simulink model "motor"  (R2015a)
settings: Solver=ode5  StartTime=0.0  StopTime=10  FixedStep=0.001  MaxStep=0.  RelTol=1e-3
undefined symbols (not defined in the file): sigbuilder_block
settings Model: Creator=Fares  LastModifiedBy=Fares

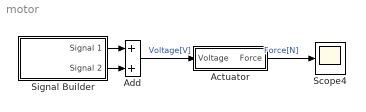
== system motor ==
  Actuator : Subsystem
  Add : Sum
  Scope4 : Scope
      settings: SaveName=ScopeData4
  Signal Builder : Subsystem  Tag=STV Subsys  LoadFcn=sigbuilder_block('load');  StartFcn=sigbuilder_block('start');  StopFcn=sigbuilder_block('stop');  ClipboardFcn=sigbuilder_block('clipboard');  mask(Sigbuilder block){}
      mask help: Simulink:masks:SigbuilderBlock_MD
      mask init:
      | if ~strcmp(get_param(bdroot(gcbh),'SimulationStatus'),'stopped') tuvar = sigbuilder_block('maskInit'); end
      settings: CopyFcn=sigbuilder_block('copy');  DeleteFcn=sigbuilder_block('delete');  ModelCloseFcn=sigbuilder_block('modelClose');  PreSaveFcn=sigbuilder_block('preSave');  PauseFcn=sigbuilder_block('pause');  ContinueFcn=sigbuilder_block('continue');  NameChangeFcn=sigbuilder_block('namechange');  OpenFcn=sigbuilder_block('open',[437.6 199.2 550.4 400 ]);  CloseFcn=sigbuilder_block('close');
      mask Display: plot(0, 0, 100, 100,[2, 2, 32, 32, 2], [68, 8, 8, 68, 68],[32, 2], [38, 38], [32, 19, 2],[53, 60, 44], [32, 17, 17, 2],[16, 16, 31, 31]);txt = getActiveGroup(gcbh);text(2, 100, txt,'verticalAlignment', 'top');
  wires:
  Actuator/1(Force) -> Scope4/1  "Force[N]"
  Signal Builder/1(Signal 1) -> Add/1
  Add/1 -> Actuator/1(Voltage)  "Voltage[V]"
  Signal Builder/2(Signal 2) -> Add/2

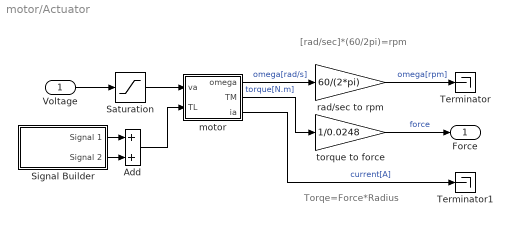
== system motor/Actuator ==
  note: Torqe=Force*Radius
  note: [rad/sec]*(60/2pi)=rpm
  Voltage : Inport
  Add : Sum
  Saturation : Saturate  UpperLimit=25  LowerLimit=-25
  Signal Builder : Subsystem  Tag=STV Subsys  LoadFcn=sigbuilder_block('load');  StartFcn=sigbuilder_block('start');  StopFcn=sigbuilder_block('stop');  ClipboardFcn=sigbuilder_block('clipboard');  mask(Sigbuilder block){}
      mask help: Simulink:masks:SigbuilderBlock_MD
      mask init:
      | if ~strcmp(get_param(bdroot(gcbh),'SimulationStatus'),'stopped') tuvar = sigbuilder_block('maskInit'); end
      settings: CopyFcn=sigbuilder_block('copy');  DeleteFcn=sigbuilder_block('delete');  ModelCloseFcn=sigbuilder_block('modelClose');  PreSaveFcn=sigbuilder_block('preSave');  PauseFcn=sigbuilder_block('pause');  ContinueFcn=sigbuilder_block('continue');  NameChangeFcn=sigbuilder_block('namechange');  OpenFcn=sigbuilder_block('open',[437.6 199.2 550.4 400 ]);  CloseFcn=sigbuilder_block('close');
      mask Display: plot(0, 0, 100, 100,[2, 2, 32, 32, 2], [68, 8, 8, 68, 68],[32, 2], [38, 38], [32, 19, 2],[53, 60, 44], [32, 17, 17, 2],[16, 16, 31, 31]);txt = getActiveGroup(gcbh);text(2, 100, txt,'verticalAlignment', 'top');
  Terminator : Terminator
  Terminator1 : Terminator
  motor : Subsystem  mask{J=140e-7, F=0.001076923, Ke=0.052, Kt=0.052, Ra=2.5, La=2.5e-3}
      mask prompts: J "Moment of inertia of the rotor [Kg.m2]"; F "Motor viscous friction constant [N.m.s]"; Ke "Electromotive force constant [V/rad/sec]"; Kt "Motor torque constant [N.m/Amp]"; Ra "Electric resistance [ohm]"; La "Electric inductance [H]"
  rad/sec to rpm : Gain  Gain=60/(2*pi)
  torque to force : Gain  Gain=1/0.0248
  Force : Outport
  wires:
  rad/sec to rpm/1 -> Terminator/1  "omega[rpm]"
  Add/1 -> motor/2(TL)
  Voltage/1 -> Saturation/1
  motor/1(omega) -> rad/sec to rpm/1  "omega[rad/s]"
  Saturation/1 -> motor/1(va)
  motor/2(TM) -> torque to force/1  "torque[N.m]"
  torque to force/1 -> Force/1  "force"
  motor/3(ia) -> Terminator1/1  "current[A]"
  Signal Builder/1(Signal 1) -> Add/1
  Signal Builder/2(Signal 2) -> Add/2

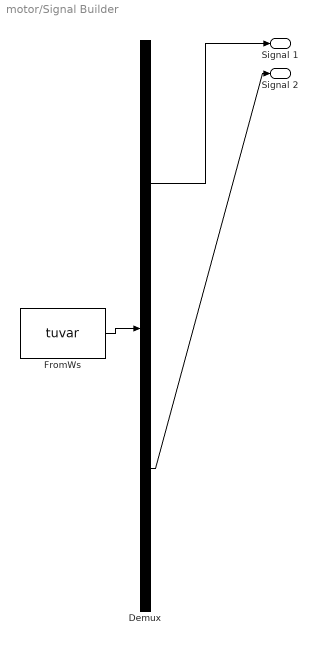
== system motor/Signal Builder ==
  Demux : Demux  Tag=STV Demux  Outputs=2
  FromWs : FromWorkspace  Tag=STV FromWs  VariableName=tuvar  SampleTime=0
      SigBuilderData=|
      | common.afterFinalStr = 'Extrapolate'
      | common.sampleTime = 0
      | dataSet.timeRange = [0 10]
      | dataSet.name = 'Group 1'
      | sbobj.Groups.Name = 'Group 1'
      | sbobj.Groups.Signals(1).Name = 'Signal 1'
      | sbobj.Groups.Signals(1).XData = [0 1 1 5 5 10]
      | sbobj.Groups.Signals(1).YData = [0 0 24 24 0 0]
      | sbobj.Groups.Signals(2).Name = 'Signal 2'
      | sbobj.Groups.Signals(2).XData = [0 6 6 10]
      | sbobj.Groups.Signals(2).YData = [0 0 -24 -24]
  Signal 1 : Outport  Tag=STV Outport
  Signal 2 : Outport  Tag=STV Outport  Port=2
  wires:
  Demux/1 -> Signal 1/1
  FromWs/1 -> Demux/1
  Demux/2 -> Signal 2/1

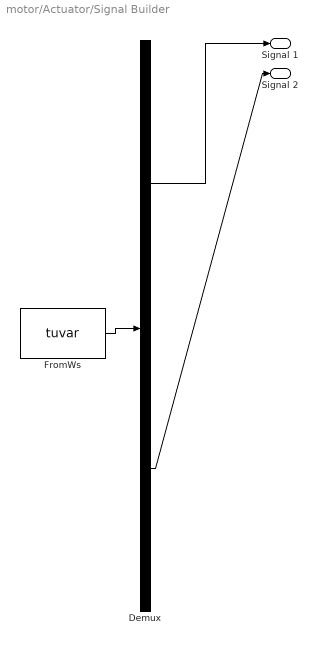
== system motor/Actuator/Signal Builder ==
  Demux : Demux  Tag=STV Demux  Outputs=2
  FromWs : FromWorkspace  Tag=STV FromWs  VariableName=tuvar  SampleTime=0
      SigBuilderData=|
      | common.afterFinalStr = 'Extrapolate'
      | common.sampleTime = 0
      | dataSet.timeRange = [0 10]
      | dataSet.name = 'Group 1'
      | sbobj.Groups.Name = 'Group 1'
      | sbobj.Groups.Signals(1).Name = 'Signal 1'
      | sbobj.Groups.Signals(1).XData = [0 3 3 5 5 10]
      | sbobj.Groups.Signals(1).YData = [0 0 0.1 0.1 0 0]
      | sbobj.Groups.Signals(2).Name = 'Signal 2'
      | sbobj.Groups.Signals(2).XData = [0 8 8 10]
      | sbobj.Groups.Signals(2).YData = [0 0 -0.1 -0.1]
  Signal 1 : Outport  Tag=STV Outport
  Signal 2 : Outport  Tag=STV Outport  Port=2
  wires:
  Demux/1 -> Signal 1/1
  FromWs/1 -> Demux/1
  Demux/2 -> Signal 2/1

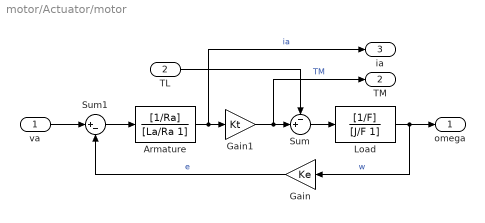
== system motor/Actuator/motor ==
  va : Inport
  TL : Inport  Port=2
  Armature : TransferFcn  Numerator=[1/Ra]  Denominator=[La/Ra 1]
  Gain : Gain  Gain=Ke
  Gain1 : Gain  Gain=Kt
  Load : TransferFcn  Numerator=[1/F]  Denominator=[J/F 1]
  Sum : Sum  Inputs=-+|
  Sum1 : Sum  Inputs=|+-
  omega : Outport
  TM : Outport  Port=2
  ia : Outport  Port=3
  wires:
  Sum/1 -> Load/1
  va/1 -> Sum1/1
  Gain/1 -> Sum1/2  "e"
  TL/1 -> Sum/1
  Gain1/1 -> TM/1, Sum/2  "TM"
  Armature/1 -> ia/1, Gain1/1  "ia"
  Load/1 -> omega/1, Gain/1  "w"
  Sum1/1 -> Armature/1
